simulink model "factorial"  (R2018a)
settings: Solver=FixedStepDiscrete  StartTime=0.0  StopTime=10.0  RelTol=1e-3  EnableMultiTasking=on
settings Model: Creator=Fady  LastModifiedBy=Fady
settings OptimizationCC: DefaultParameterBehavior=Inlined  InlineInvariantSignals=on  EnableMemcpy=off  LifeSpan=1
settings DebuggingCC: UnderspecifiedInitializationDetection=Classic  MergeDetectMultiDrivingBlocksExec=none
settings ModelReferenceCC: PropagateSignalLabelsOutOfModel=off
settings SFSimCC: MATLABDynamicMemAlloc=off
settings RTWCC: SystemTargetFile=ert.tlc  GenCodeOnly=on  TemplateMakefile=ert_default_tmf  GenerateReport=on  IncludeHyperlinkInReport=on  LaunchReport=on  GenerateTraceInfo=on  GenerateTraceReport=on  GenerateTraceReportSl=on  GenerateTraceReportSf=on  GenerateTraceReportEml=on
settings CodeAppCC: ForceParamTrailComments=on  IgnoreCustomStorageClasses=off  OperatorAnnotations=on  SimulinkDataObjDesc=on  SFDataObjDesc=on  MATLABFcnDesc=on  InsertBlockDesc=on  StateflowObjectComments=on  MATLABSourceComments=on
settings ERTTargetCC: MultiwordLength=2048  GenerateSampleERTMain=on  InlinedParameterPlacement=NonHierarchical  ERTCustomFileTemplate=example_file_process.tlc

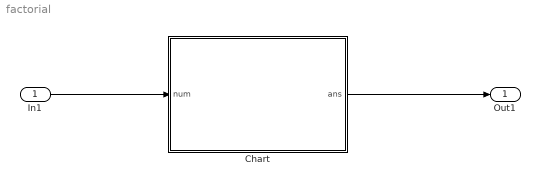
== system factorial ==
  In1 : Inport  OutDataTypeStr=uint8
  Chart : Stateflow chart  TreatAsAtomicUnit=on
  Out1 : Outport  OutDataTypeStr=uint32
  wires:
  In1/1 -> Chart/1(num)
  Chart/1(ans) -> Out1/1

== stateflow chart factorial/Chart ==
  (default) -> (junction 8) : % Factorial
      | {ans=1;}
  (junction 9) -> (junction 7) [order 1] : [i<=num]
  (junction 7) -> (junction 10) : {ans=ans*i;}
  (junction 8) -> (junction 9) : {i=1;}
  (junction 10) -> (junction 9) : {i=i+1;}
  (junction 9) -> (junction 11) [order 2]
  data: ans output uint32; num input uint8; i local uint8
